simulink library "Storage_Type_1_CONF"  (R2016b)
settings: Solver=ode45  StartTime=0.0  StopTime=10.0  RelTol=1e-3  EnableMultiTasking=on
undefined symbols (not defined in the file): path_carnot
libraries: carnot x6
settings Model: Creator=lena.frank  LastModifiedBy=drhf
settings DataIOCC: LimitDataPoints=on  SaveFormat=Array  SignalLoggingSaveFormat=ModelDataLogs
settings OptimizationCC: ExpressionDepthLimit=2147483647  LifeSpan=inf
settings DebuggingCC: UnderspecifiedInitializationDetection=Classic  MergeDetectMultiDrivingBlocksExec=none  SolverPrmCheckMsg=warning  FcnCallInpInsideContextMsg=warning  StateNameClashWarn=warning  SFUnexpectedBacktrackingDiag=warning  SFNoUnconditionalDefaultTransitionDiag=warning  SFExecutionAtInitializationDiag=none
settings HardwareCC: ProdBitPerPointer=32  ProdBitPerSizeT=32  ProdBitPerPtrDiffT=32  ProdLargestAtomicFloat=None  ProdIntDivRoundTo=Undefined  ProdEndianess=Unspecified  ProdWordSize=32  ProdHWDeviceType=32-bit Generic
settings ModelReferenceCC: PropagateSignalLabelsOutOfModel=off
settings GRTTargetCC: TargetLangStandard=C89/C90 (ANSI)  GeneratePreprocessorConditionals=Disable all  CombineOutputUpdateFcns=off  GRTInterface=on
settings ConfigComp: CovMetricSettings=dw  CovHtmlReporting=on  CovSaveCumulativeToWorkspaceVar=on  CovSaveSingleToWorkspaceVar=on  CovExternalEMLEnable=off

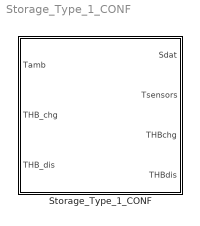
== system Storage_Type_1_CONF ==
  Storage_Type_1_CONF : Subsystem  mask(Buffer storage tank){t0=[10:5:55], hgt=1.7684, stgtype=1, tini=[10 15 20 25 30 35 40 45 50 55], mpts=[1 2 3 4 5 6 7 8 9 10], PathName=fullfile(path_carnot('libsl'),'Storage','Thermal','Storage_Type_1_CONF','parameter_set'), FileName='StorageType1_500_L.mat', userPath=off, userParam=off, uwall=1, ubot=1, utop=1, axcond=1, volume=0.5, dia=0.6, standing=standing cylinder, nodes=10, mpoints=10, Tsensor=0.5, pipe1inlet=1, pipe1outlet=0, pipe1dia=0.03, pipe2inlet=0, pipe2outlet=1, pipe2dia=0.03}
      mask prompts: t0 "Initial temperature (vector or scalar) in °C"; hgt "Height of storage in m"; stgtype "Storage Type (0..5)"; tini "Start temperatures of nodes in °C"; mpts "Index to measured nodes"; PathName "Path"; FileName "Parameter set"; userPath "Edit path and name of parameter set"; userParam "User defined parameters"; uwall "Heat transfer coefficient to ambient [W/m²K]"; ubot "Heat transfer coefficient to ambient bottom [W/m²K]"; utop "Heat transfer coefficient to ambient top [W/m²K]"; axcond "Effective thermal conductivity [W/m/K]"; volume "Volume [m³]"; dia "Diameter [m]"; standing "Position"; nodes "Number of nodes"; mpoints "Number of node temperatures (for display)"; Tsensor "Temperature sensor position (0..1, 0 = bottom, 1 = top)"; pipe1inlet "relative height of inlet, range from 0 (= bottom) to 1 (= top)"; pipe1outlet "relative height of outlet, range from 0 (= bottom) to 1 (= top)"; pipe1dia "Diameter of pipe in m"; pipe2inlet "relative height of inlet, range from 0 (= bottom) to 1 (= top)"; pipe2outlet "relative height of outlet, range from 0 (= bottom) to 1 (= top)"; pipe2dia "Diameter of pipe in m"
      mask help:
      | Buffer storage for heating circuits. The storage model has the following components (with their typical position):
      | - one pipe connection for discharging (total height)
      | - one pipe connection for charging (total height)
      mask init:
      | [ok, param] = CarnotCallbacks_StorageConf('SetParam',stgtype,gcbh,PathName,FileName);
      mask Help: web(fullfile(path_carnot('help'),'Storage_Type_N.html'),'-helpbrowser')
      mask TypeOptions hgt: Pipe_Connection_1/hgt | Pipe_Connection_2/hgt
      mask TypeOptions stgtype: CreateSdat/stgtype
      mask TypeOptions tini: sfun_storageTnodes/tini
      mask TypeOptions mpts: select_T/Indices
      mask Callback userPath: [ok, param] = CarnotCallbacks_StorageConf('UserEdit',1,gcbh);
      mask Callback userParam: [ok, param] = CarnotCallbacks_StorageConf('UserEdit',1,gcbh);
      mask TypeOptions uwall: sfun_storageTnodes/uloss
      mask TypeOptions ubot: sfun_storageTnodes/ubot
      mask TypeOptions utop: sfun_storageTnodes/utop
      mask TypeOptions axcond: sfun_storageTnodes/cond
      mask TypeOptions volume: sfun_storageTnodes/volume | CreateSdat/volume
      mask TypeOptions dia: sfun_storageTnodes/dia
      mask TypeOptions standing: sfun_storageTnodes/standing
      mask TypeOptions nodes: sfun_storageTnodes/nodes | select_T/InputPortWidth | HX_EN12977_1/nodes | HX_EN12977_2/nodes | HX_EN12977_3/nodes | Pipe_Connection_1/nodes | Pipe_Connection_2/nodes | Pipe_Connection_3/nodes
      mask TypeOptions Tsensor: T_Sensor_Surface/pos
      mask TypeOptions pipe1inlet: Pipe_Connection_1/h_in
      mask TypeOptions pipe1outlet: Pipe_Connection_1/h_out
      mask TypeOptions pipe1dia: Pipe_Connection_1/dia
      mask TypeOptions pipe2inlet: Pipe_Connection_2/h_in
      mask TypeOptions pipe2outlet: Pipe_Connection_2/h_out
      mask TypeOptions pipe2dia: Pipe_Connection_2/dia
      mask DialogControl Container14 Prompt: Infos
      mask DialogControl Control3 Prompt: Carnot public data
      mask DialogControl Control3 Callback: [ok, file] = CarnotCallbacks_StorageConf('GetFilename',1,gcbh,'public');
      mask DialogControl Control4 Prompt: Carnot internal data
      mask DialogControl Control4 Callback: [ok, file] = CarnotCallbacks_StorageConf('GetFilename',1,gcbh,'internal');
      mask DialogControl Control2 Prompt: Selected path
      mask DialogControl Control2 Callback: [ok, file] = CarnotCallbacks_StorageConf('GetFilename',1,gcbh,'selected');
      mask DialogControl Control6 Prompt: Save in Carnot internal data
      mask DialogControl Control6 Callback: [ok, param] = CarnotCallbacks_StorageConf('SaveFilename',1,gcbh,'internal','STG');
      mask DialogControl Control5 Prompt: Save in selected path
      mask DialogControl Control5 Callback: [ok, param] = CarnotCallbacks_StorageConf('SaveFilename',1,gcbh,'selected','STG');
      mask Display:
      | % user defined picture file
      | namestr = ['Storage_Type_', num2str(get_param(gcb,'stgtype'))];
      | picfile = fullfile(path_carnot('intlibsl'), 'Storage','Thermal', ...
      |     namestr,'parameter_set', [namestr, '.jpg']);
      | 
      | % show public picture
      | plot([40,40,45,55,60,60,55,45,40]/100,[84,36,30,30,36,84,90,90,84]/100, ...
      |     [40,35]/100,[77,77]/100,[64,60]/100,[77,77]/100,[40,35]/100,[42,42]/100, ...
      |     [64,60]/100,[42,42]/100)
      | set_param(gcb, 'BackgroundColor', 'Red')
      | 
      | % show internal picture if defined
      | if  ~BlockIsInCarnotLibrary       % if not located in library
      |     if exist(picfile, 'file')
      |         image(imread(picfile), [0.25, 0, 0.45, 1])
      |         set_param(gcb, 'BackgroundColor', 'White')
      |     end
      | end

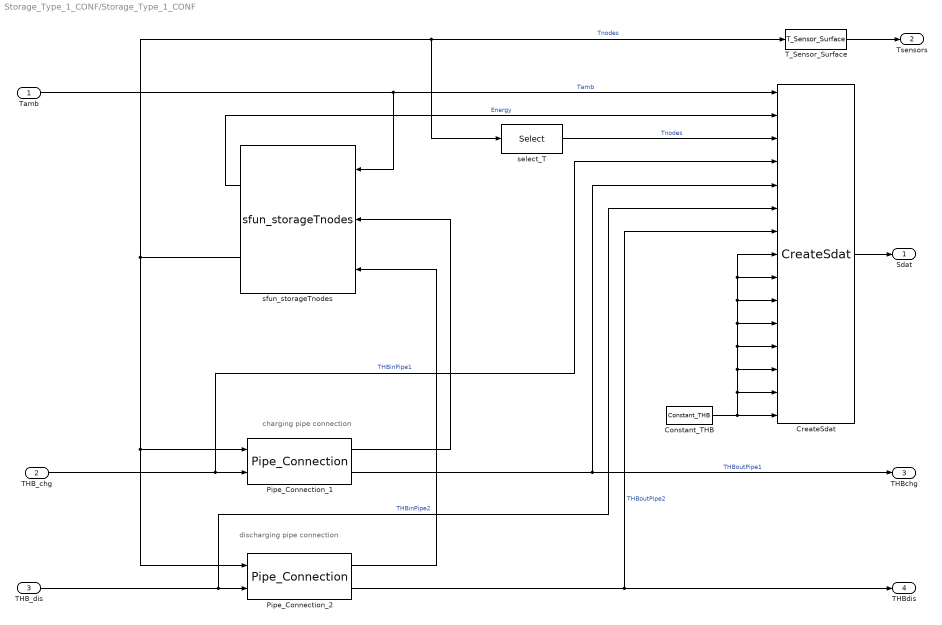
== system Storage_Type_1_CONF/Storage_Type_1_CONF ==
  note: discharging pipe connection
  note: charging pipe connection
  Tamb : Inport
  THB_chg : Inport  Port=2
  THB_dis : Inport  Port=3
  Constant_THB : carnot/Source/Simple/Constant_THB  t=20  mdot=0  p=1e5  mID=No Pressure Drop  fluid=Water  mix=0  mix2=0  mix3=0  dia=0.02  hgt=0
  CreateSdat : carnot/Basic/Thermal_Models/CreateSdat  volume=volume  stgtype=stgtype
  Pipe_Connection_1 : carnot/Storage/Thermal/Storage_Ports/Pipe_Connection  h_in=pipe1inlet  h_out=pipe1outlet  hgt=hgt  dia=pipe1dia  height=-1.7684  nodes=nodes
  Pipe_Connection_2 : carnot/Storage/Thermal/Storage_Ports/Pipe_Connection  h_in=pipe2inlet  h_out=pipe2outlet  hgt=hgt  dia=pipe2dia  height=1.7684  nodes=nodes
  T_Sensor_Surface : carnot/Control/T_Sensor_Surface  pos=Tsensor  tdel=10  t0=mean(tini)
  select_T : Selector  InputPortWidth=nodes  IndexOptions=Index vector (dialog)  Indices=[1 2 3 4 5 6 7 8 9 10]  OutputSizes=1
  sfun_storageTnodes : carnot/Basic/Thermal_Models/sfun_storageTnodes  uloss=uwall  ubot=ubot  utop=utop  cond=axcond  volume=volume  dia=dia  standing=standing cylinder  tini=tini  nodes=nodes  nconnect=2  elimthermocline=2  condinvtc=1e5
  Sdat : Outport
  Tsensors : Outport  Port=2
  THBchg : Outport  Port=3
  THBdis : Outport  Port=4
  wires:
  Constant_THB/1 -> CreateSdat/15, CreateSdat/8, CreateSdat/9, CreateSdat/10, CreateSdat/11, CreateSdat/12, CreateSdat/13, CreateSdat/14
  T_Sensor_Surface/1 -> Tsensors/1
  Pipe_Connection_1/1 -> sfun_storageTnodes/2
  Pipe_Connection_1/2 -> THBchg/1, CreateSdat/5  "THBoutPipe1"
  THB_chg/1 -> Pipe_Connection_1/2, CreateSdat/4  "THBinPipe1"
  CreateSdat/1 -> Sdat/1
  sfun_storageTnodes/2 -> Pipe_Connection_1/1, Pipe_Connection_2/1, T_Sensor_Surface/1, select_T/1  "Tnodes"
  select_T/1 -> CreateSdat/3  "Tnodes"
  Tamb/1 -> CreateSdat/1, sfun_storageTnodes/1  "Tamb"
  THB_dis/1 -> CreateSdat/6, Pipe_Connection_2/2  "THBinPipe2"
  Pipe_Connection_2/1 -> sfun_storageTnodes/3
  Pipe_Connection_2/2 -> THBdis/1, CreateSdat/7  "THBoutPipe2"
  sfun_storageTnodes/1 -> CreateSdat/2  "Energy"
